simulink model "lab5_EAs"  (R2021b)
settings: Solver=VariableStepAuto  StartTime=0.0  StopTime=10.0  RelTol=1e-3
values from neighbouring files (symbols this model uses):
  J = [Ixx 0 0; 0 Iyy 0; 0 0 Izz]    [euler_equation_tasks.m]    (also in lab5_task2.m)
  Jinv = inv(J)    [euler_equation_tasks.m]    (also in lab5_task2.m)
  theta0 = deg2rad(0)    [Lab08_script.m]    (also in Lab7_script.m = deg2rad(230); Lab7_scriptscalar.m = deg2rad(230))
  w0 = [0.45 0.52 0.55]'    [euler_equation_tasks.m]    (also in lab5_task2.m = [C 0.1 0.1]')
undefined symbols (not defined in the file or in its folder): phi0, psi0
libraries: matrix_library x1
settings Model: Creator=samuz  LastModifiedBy=samuz

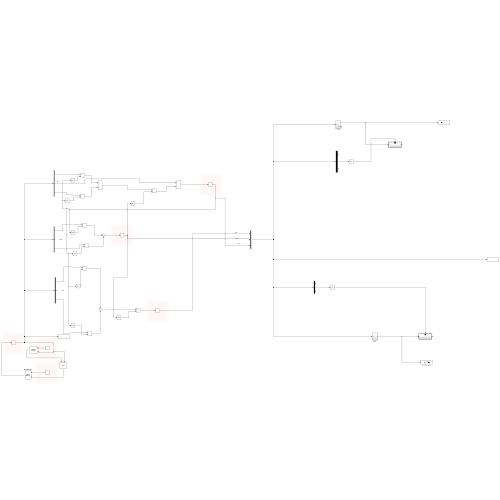
[thumbnail: Simulink's stored preview of the top-level diagram]
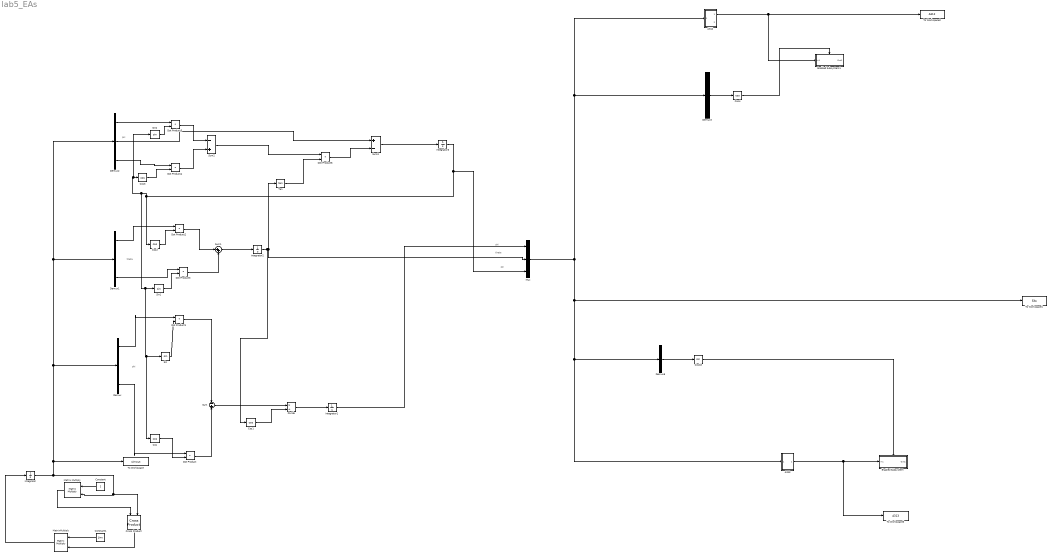
== system lab5_EAs ==
  note: psi
  note: theta
  note: phi
  note: psi
  note: theta
  note: phi
  A312 : Subsystem
  A313 : Subsystem
  Constant : Constant  Value=J
  Constant1 : Constant  Value=Jinv
  Cos{,1..4} (5 alike) : Trigonometry  Operator=cos
  Cos18 : Trigonometry
  Cross Product : matrix_library/Cross Product
      settings: SourceProductBaseCode=SL
  Demux{,1..3,6} (5 alike) : Demux  Outputs=3
  Divide : Product  Inputs=*/
  Dot Product{,1..6} (7 alike) : DotProduct  InputSameDT=on  OutDataTypeStr=Inherit: Inherit via internal rule
  Enabled Subsystem : Subsystem  TreatAsAtomicUnit=on
  Enabled Subsystem1 : Subsystem  TreatAsAtomicUnit=on
  Integrator : Integrator  InitialCondition=w0
  Integrator1 : Integrator  InitialCondition=phi0
  Integrator2 : Integrator  InitialCondition=theta0
  Integrator3 : Integrator  InitialCondition=psi0
  Matrix Multiply : Product  Multiplication=Matrix(*)
  MatrixMultiply : Product  Multiplication=Matrix(*)
  Mux : Mux  Inputs=3
  Sin : Trigonometry
  Sin1 : Trigonometry
  Sin2 : Trigonometry
  Sum : Sum  Inputs=-+
  Sum1 : Sum  Inputs=|++
  Sum2 : Sum  Inputs=-+
  Sum3 : Sum  Inputs=+-
  Tan : Trigonometry  Operator=tan
  To Workspace : ToWorkspace  VariableName=simout  SampleTime=-1
  To Workspace1 : ToWorkspace  VariableName=EAs  SampleTime=-1
  To Workspace2 : ToWorkspace  VariableName=A312  SaveFormat=Timeseries  SampleTime=-1
  To Workspace3 : ToWorkspace  VariableName=A313  SaveFormat=Timeseries  SampleTime=-1
  wires:
  Cross Product/1 -> MatrixMultiply/2
  Matrix Multiply/1 -> Cross Product/1
  Integrator/1 -> To Workspace/1, Demux2/1, Demux1/1, Demux/1, Cross Product/2, Matrix Multiply/2
  MatrixMultiply/1 -> Integrator/1
  Constant1/1 -> MatrixMultiply/1
  Constant/1 -> Matrix Multiply/1
  Demux/3 -> Dot Product/1
  Cos/1 -> Dot Product/2
  Demux/1 -> Dot Product1/1
  Sin/1 -> Dot Product1/2
  Dot Product1/1 -> Sum/1
  Dot Product/1 -> Sum/2
  Sum/1 -> Divide/1
  Cos1/1 -> Divide/2
  Divide/1 -> Integrator1/1
  Cos2/1 -> Dot Product2/2
  Sin1/1 -> Dot Product3/2
  Demux1/1 -> Dot Product2/1
  Demux1/3 -> Dot Product3/1
  Dot Product2/1 -> Sum1/1
  Dot Product3/1 -> Sum1/2
  Sum1/1 -> Integrator2/1
  Demux2/3 -> Dot Product4/1
  Cos3/1 -> Dot Product4/2
  Sin2/1 -> Dot Product5/2
  Demux2/1 -> Dot Product5/1
  Dot Product4/1 -> Sum2/2
  Dot Product5/1 -> Sum2/1
  Integrator2/1 -> Mux/2, Tan/1, Cos1/1
  Sum2/1 -> Dot Product6/1
  Tan/1 -> Dot Product6/2
  Dot Product6/1 -> Sum3/2
  Demux2/2 -> Sum3/1
  Sum3/1 -> Integrator3/1
  Integrator3/1 -> Cos/1, Sin/1, Sin1/1, Sin2/1, Cos3/1, Cos2/1, Mux/3
  Integrator1/1 -> Mux/1
  Mux/1 -> Demux3/1, A312/1(In1), Demux6/1, A313/1(In1), To Workspace1/1
  A313/1(Out1) -> Enabled Subsystem/1(In1), To Workspace3/1
  Demux6/2 -> Cos18/1
  Cos18/1 -> Enabled Subsystem/Enable
  A312/1(Out1) -> Enabled Subsystem1/1(In1), To Workspace2/1
  Demux3/2 -> Cos4/1
  Cos4/1 -> Enabled Subsystem1/Enable

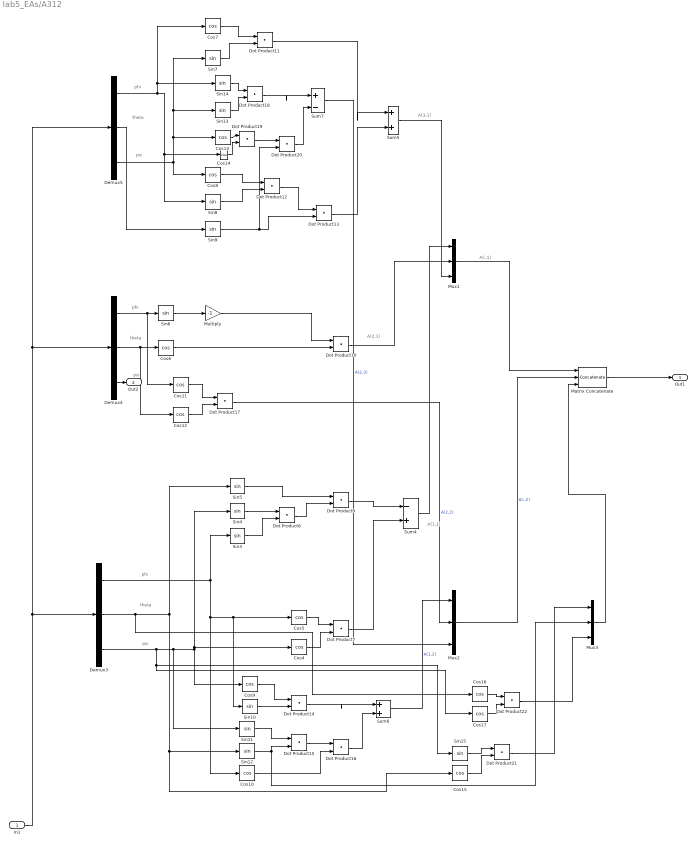
== system lab5_EAs/A312 ==
  note: A(:,1)
  note: A(3,1)
  note: A(2,1)
  note: A(1,1)
  note: psi
  note: psi
  note: theta
  note: phi
  note: phi
  note: theta
  note: psi
  note: phi
  note: theta
  In1 : Inport
  Cos{4..17} (14 alike) : Trigonometry  Operator=cos
  Demux3 : Demux  Outputs=3
  Demux4 : Demux  Outputs=3
  Demux5 : Demux  Outputs=3
  Dot Product{7..22} (16 alike) : DotProduct  InputSameDT=on  OutDataTypeStr=Inherit: Inherit via internal rule
  Matrix Concatenate : Concatenate  NumInputs=3  Mode=Multidimensional array  ConcatenateDimension=2
  Multiply : Gain  Gain=-1
  Mux1 : Mux  Inputs=3
  Mux2 : Mux  Inputs=3
  Mux3 : Mux  Inputs=3
  Sin{3..15} (13 alike) : Trigonometry
  Sum4 : Sum  Inputs=-+
  Sum5 : Sum  Inputs=|++
  Sum6 : Sum  Inputs=|++
  Sum7 : Sum  Inputs=|+-
  Out1 : Outport
  Out2 : Outport  Port=2
  wires:
  Cos15/1 -> Dot Product21/2
  Demux4/1 -> Cos11/1, Sin6/1
  Demux3/3 -> Cos17/1, Sin15/1, Sin11/1, Sin4/1, Cos4/1, Cos9/1
  Cos11/1 -> Dot Product17/1
  Sin11/1 -> Dot Product15/1
  Dot Product10/1 -> Mux1/2
  Demux5/3 -> Cos13/1, Sin7/1, Sin13/1, Cos8/1
  Sin7/1 -> Dot Product11/2
  Demux4/2 -> Cos12/1, Cos6/1
  Dot Product12/1 -> Dot Product13/1
  Dot Product7/1 -> Sum4/2
  Dot Product9/1 -> Sum4/1
  In1/1 -> Demux5/1, Demux4/1, Demux3/1
  Sin9/1 -> Dot Product20/2, Dot Product13/2
  Dot Product11/1 -> Sum5/1
  Sin10/1 -> Dot Product14/2
  Sin5/1 -> Dot Product9/1
  Dot Product15/1 -> Dot Product16/1
  Dot Product18/1 -> Sum7/1
  Sum5/1 -> Mux1/3
  Mux2/1 -> Matrix Concatenate/2  "A(:,2)"
  Demux5/1 -> Sin14/1, Cos7/1, Cos14/1, Sin8/1
  Sin3/1 -> Dot Product8/2
  Demux3/2 -> Cos16/1, Cos15/1, Sin12/1, Sin5/1
  Demux3/1 -> Cos10/1, Sin10/1, Cos5/1, Sin3/1
  Cos6/1 -> Dot Product10/2
  Cos7/1 -> Dot Product11/1
  Dot Product13/1 -> Sum5/2
  Sin6/1 -> Multiply/1
  Sin4/1 -> Dot Product8/1
  Dot Product22/1 -> Mux3/3
  Cos8/1 -> Dot Product12/1
  Multiply/1 -> Dot Product10/1
  Dot Product8/1 -> Dot Product9/2
  Demux4/3 -> Out2/1
  Cos5/1 -> Dot Product7/1
  Demux5/2 -> Sin9/1
  Sin15/1 -> Dot Product21/1
  Dot Product14/1 -> Sum6/1
  Cos10/1 -> Dot Product16/2
  Sin14/1 -> Dot Product18/1
  Sin13/1 -> Dot Product18/2
  Sum6/1 -> Mux2/1  "A(1,2)"
  Dot Product20/1 -> Sum7/2
  Sin8/1 -> Dot Product12/2
  Mux1/1 -> Matrix Concatenate/1
  Sum7/1 -> Mux2/3  "A(2,3)"
  Dot Product21/1 -> Mux3/1
  Cos12/1 -> Dot Product17/2
  Cos9/1 -> Dot Product14/1
  Sum4/1 -> Mux1/1
  Dot Product17/1 -> Mux2/2  "A(2,2)"
  Cos13/1 -> Dot Product19/1
  Cos14/1 -> Dot Product19/2
  Dot Product19/1 -> Dot Product20/1
  Cos16/1 -> Dot Product22/1
  Dot Product16/1 -> Sum6/2
  Cos4/1 -> Dot Product7/2
  Cos17/1 -> Dot Product22/2
  Sin12/1 -> Mux3/2, Dot Product15/2
  Mux3/1 -> Matrix Concatenate/3
  Matrix Concatenate/1 -> Out1/1

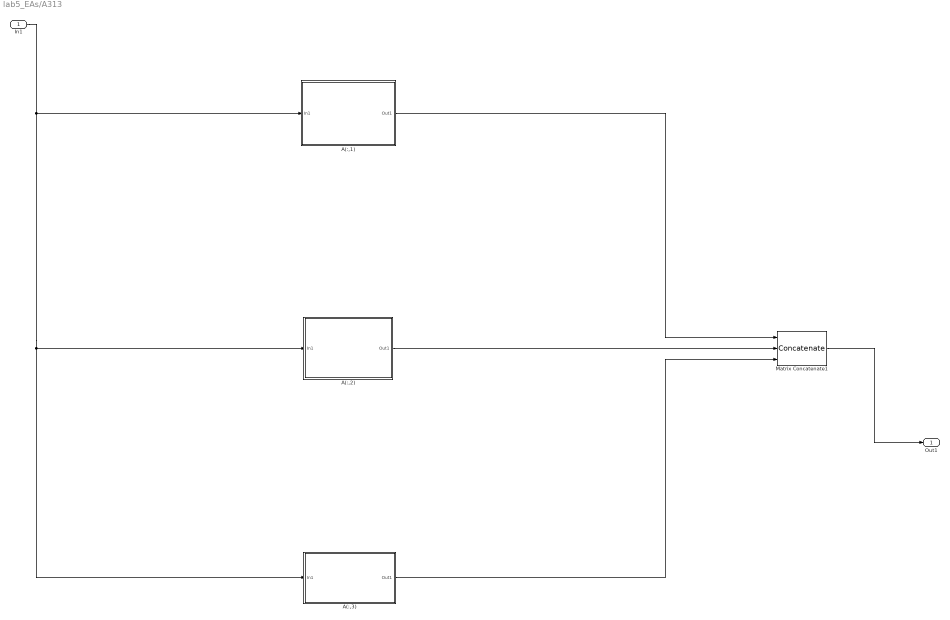
== system lab5_EAs/A313 ==
  In1 : Inport
  A(:,1) : Subsystem
  A(:,2) : Subsystem
  A(:,3) : Subsystem
  Matrix Concatenate1 : Concatenate  NumInputs=3  Mode=Multidimensional array  ConcatenateDimension=2
  Out1 : Outport
  wires:
  In1/1 -> A(:,3)/1(In1), A(:,2)/1(In1), A(:,1)/1(In1)
  A(:,3)/1(Out1) -> Matrix Concatenate1/3
  A(:,2)/1(Out1) -> Matrix Concatenate1/2
  A(:,1)/1(Out1) -> Matrix Concatenate1/1
  Matrix Concatenate1/1 -> Out1/1

== system lab5_EAs/Enabled Subsystem ==
  In1 : Inport
  Enable : EnablePort
  Out1 : Outport
  wires:
  In1/1 -> Out1/1

== system lab5_EAs/Enabled Subsystem1 ==
  In1 : Inport
  Enable : EnablePort
  Out1 : Outport
  wires:
  In1/1 -> Out1/1

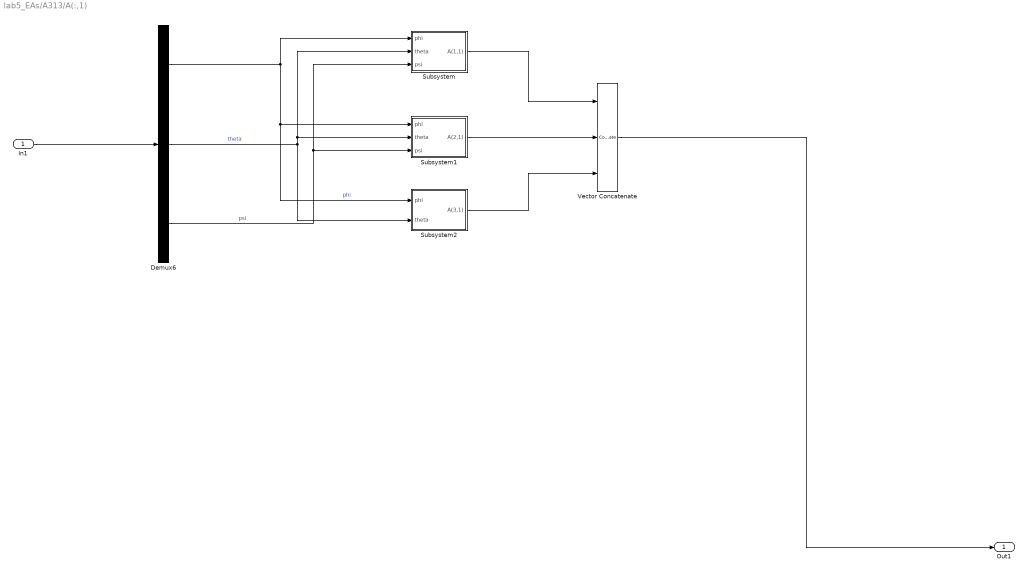
== system lab5_EAs/A313/A(:,1) ==
  In1 : Inport
  Demux6 : Demux  Outputs=3
  Subsystem : Subsystem
  Subsystem1 : Subsystem
  Subsystem2 : Subsystem
  Vector Concatenate : Concatenate  NumInputs=3
  Out1 : Outport
  wires:
  Subsystem2/1(A(3,1)) -> Vector Concatenate/3
  Demux6/1 -> Subsystem2/1(phi), Subsystem1/1(phi), Subsystem/1(phi)  "phi"
  Demux6/3 -> Subsystem1/3(psi), Subsystem/3(psi)  "psi"
  Subsystem1/1(A(2,1)) -> Vector Concatenate/2
  Demux6/2 -> Subsystem2/2(theta), Subsystem1/2(theta), Subsystem/2(theta)  "theta"
  In1/1 -> Demux6/1
  Subsystem/1(A(1,1)) -> Vector Concatenate/1
  Vector Concatenate/1 -> Out1/1

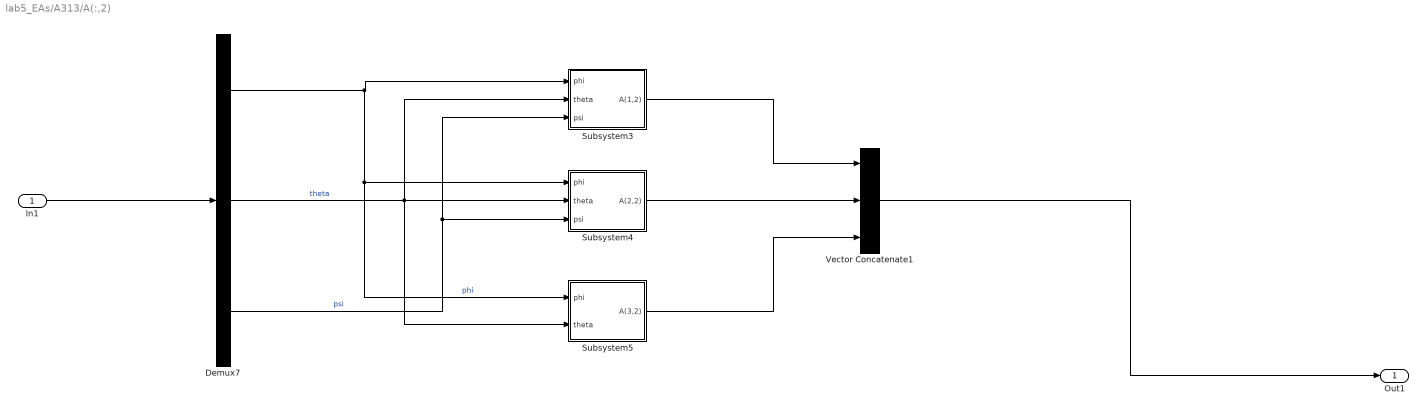
== system lab5_EAs/A313/A(:,2) ==
  In1 : Inport
  Demux7 : Demux  Outputs=3
  Subsystem3 : Subsystem
  Subsystem4 : Subsystem
  Subsystem5 : Subsystem
  Vector Concatenate1 : Concatenate  NumInputs=3
  Out1 : Outport
  wires:
  Demux7/3 -> Subsystem4/3(psi), Subsystem3/3(psi)  "psi"
  Subsystem5/1(A(3,2)) -> Vector Concatenate1/3
  In1/1 -> Demux7/1
  Subsystem4/1(A(2,2)) -> Vector Concatenate1/2
  Demux7/1 -> Subsystem3/1(phi), Subsystem5/1(phi), Subsystem4/1(phi)  "phi"
  Vector Concatenate1/1 -> Out1/1
  Demux7/2 -> Subsystem4/2(theta), Subsystem5/2(theta), Subsystem3/2(theta)  "theta"
  Subsystem3/1(A(1,2)) -> Vector Concatenate1/1

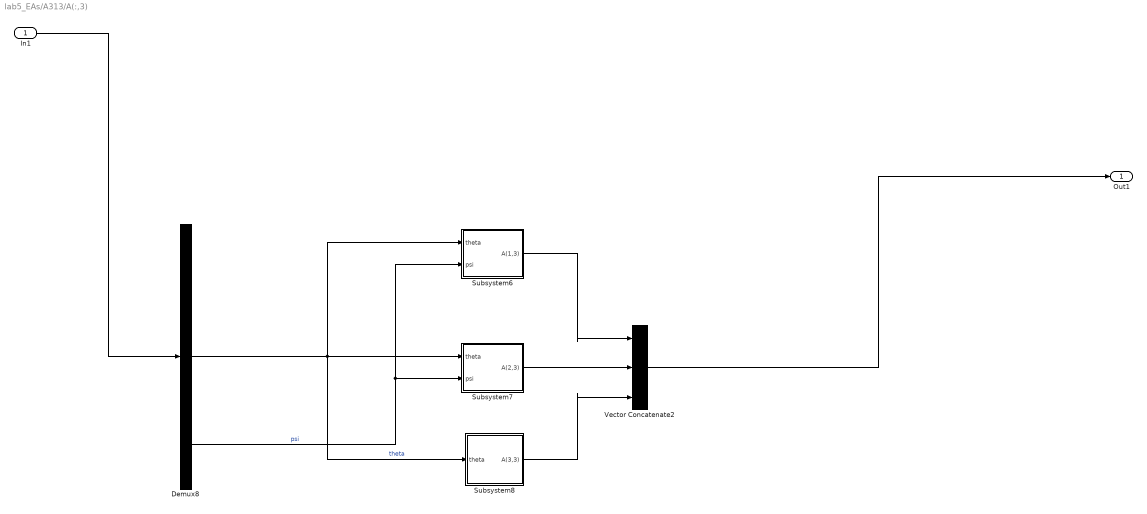
== system lab5_EAs/A313/A(:,3) ==
  In1 : Inport
  Demux8 : Demux  Outputs=3
  Subsystem6 : Subsystem
  Subsystem7 : Subsystem
  Subsystem8 : Subsystem
  Vector Concatenate2 : Concatenate  NumInputs=3
  Out1 : Outport
  wires:
  Demux8/2 -> Subsystem8/1(theta), Subsystem6/1(theta), Subsystem7/1(theta)  "theta"
  Subsystem7/1(A(2,3)) -> Vector Concatenate2/2
  Vector Concatenate2/1 -> Out1/1
  Subsystem8/1(A(3,3)) -> Vector Concatenate2/3
  Subsystem6/1(A(1,3)) -> Vector Concatenate2/1
  In1/1 -> Demux8/1
  Demux8/3 -> Subsystem7/2(psi), Subsystem6/2(psi)  "psi"

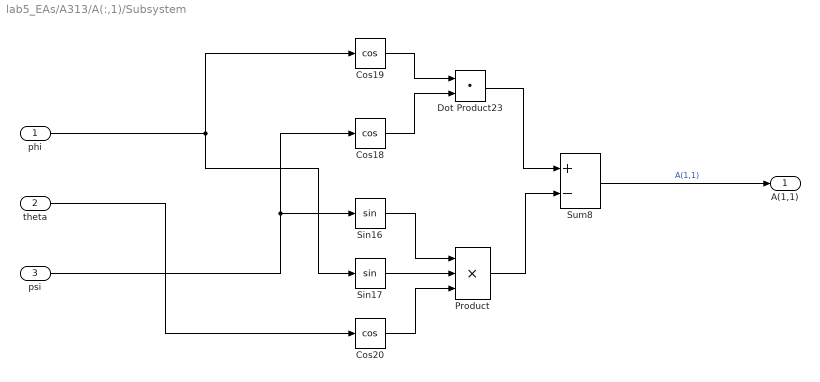
== system lab5_EAs/A313/A(:,1)/Subsystem ==
  phi : Inport
  theta : Inport  Port=2
  psi : Inport  Port=3
  Cos18 : Trigonometry  Operator=cos
  Cos19 : Trigonometry  Operator=cos
  Cos20 : Trigonometry  Operator=cos
  Dot Product23 : DotProduct  InputSameDT=on  OutDataTypeStr=Inherit: Inherit via internal rule
  Product : Product  Inputs=3
  Sin16 : Trigonometry
  Sin17 : Trigonometry
  Sum8 : Sum  Inputs=+-
  A(1,1) : Outport
  wires:
  psi/1 -> Sin16/1, Cos18/1
  Dot Product23/1 -> Sum8/1
  Sin16/1 -> Product/1
  Cos18/1 -> Dot Product23/2
  Sin17/1 -> Product/2
  Cos19/1 -> Dot Product23/1
  Product/1 -> Sum8/2
  Sum8/1 -> A(1,1)/1  "A(1,1)"
  Cos20/1 -> Product/3
  phi/1 -> Cos19/1, Sin17/1
  theta/1 -> Cos20/1

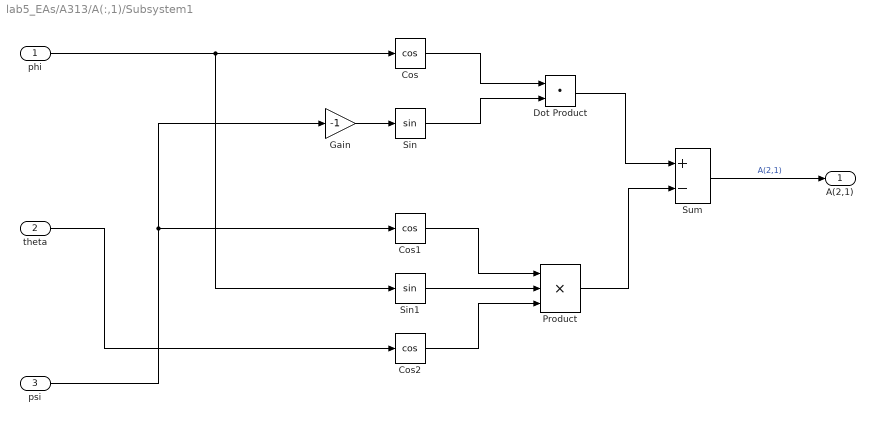
== system lab5_EAs/A313/A(:,1)/Subsystem1 ==
  phi : Inport
  theta : Inport  Port=2
  psi : Inport  Port=3
  Cos : Trigonometry  Operator=cos
  Cos1 : Trigonometry  Operator=cos
  Cos2 : Trigonometry  Operator=cos
  Dot Product : DotProduct  InputSameDT=on  OutDataTypeStr=Inherit: Inherit via internal rule
  Gain : Gain  Gain=-1
  Product : Product  Inputs=3
  Sin : Trigonometry
  Sin1 : Trigonometry
  Sum : Sum  Inputs=+-
  A(2,1) : Outport
  wires:
  psi/1 -> Cos1/1, Gain/1
  phi/1 -> Cos/1, Sin1/1
  Gain/1 -> Sin/1
  Cos/1 -> Dot Product/1
  Sin/1 -> Dot Product/2
  theta/1 -> Cos2/1
  Cos1/1 -> Product/1
  Sin1/1 -> Product/2
  Cos2/1 -> Product/3
  Dot Product/1 -> Sum/1
  Product/1 -> Sum/2
  Sum/1 -> A(2,1)/1  "A(2,1)"

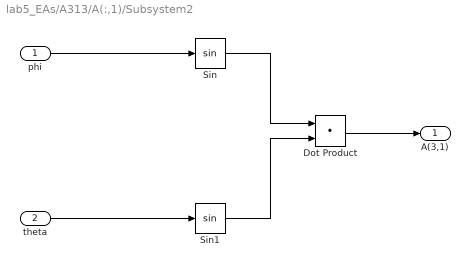
== system lab5_EAs/A313/A(:,1)/Subsystem2 ==
  phi : Inport
  theta : Inport  Port=2
  Dot Product : DotProduct  InputSameDT=on  OutDataTypeStr=Inherit: Inherit via internal rule
  Sin : Trigonometry
  Sin1 : Trigonometry
  A(3,1) : Outport
  wires:
  phi/1 -> Sin/1
  theta/1 -> Sin1/1
  Sin/1 -> Dot Product/1
  Sin1/1 -> Dot Product/2
  Dot Product/1 -> A(3,1)/1

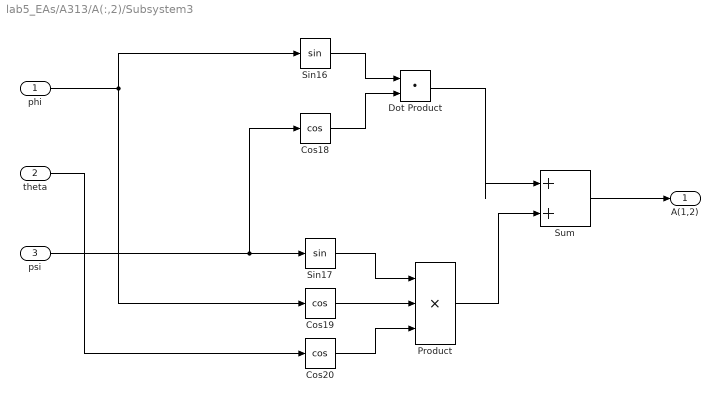
== system lab5_EAs/A313/A(:,2)/Subsystem3 ==
  phi : Inport
  theta : Inport  Port=2
  psi : Inport  Port=3
  Cos18 : Trigonometry  Operator=cos
  Cos19 : Trigonometry  Operator=cos
  Cos20 : Trigonometry  Operator=cos
  Dot Product : DotProduct  InputSameDT=on  OutDataTypeStr=Inherit: Inherit via internal rule
  Product : Product  Inputs=3
  Sin16 : Trigonometry
  Sin17 : Trigonometry
  Sum : Sum  Inputs=|++
  A(1,2) : Outport
  wires:
  Cos18/1 -> Dot Product/2
  phi/1 -> Cos19/1, Sin16/1
  psi/1 -> Cos18/1, Sin17/1
  Sin16/1 -> Dot Product/1
  theta/1 -> Cos20/1
  Sin17/1 -> Product/1
  Cos19/1 -> Product/2
  Cos20/1 -> Product/3
  Dot Product/1 -> Sum/1
  Product/1 -> Sum/2
  Sum/1 -> A(1,2)/1

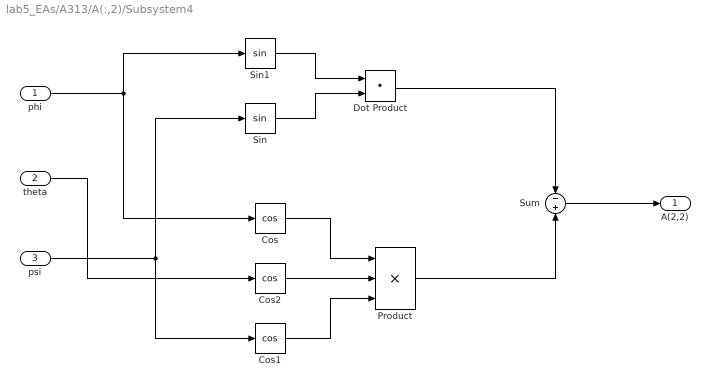
== system lab5_EAs/A313/A(:,2)/Subsystem4 ==
  phi : Inport
  theta : Inport  Port=2
  psi : Inport  Port=3
  Cos : Trigonometry  Operator=cos
  Cos1 : Trigonometry  Operator=cos
  Cos2 : Trigonometry  Operator=cos
  Dot Product : DotProduct  InputSameDT=on  OutDataTypeStr=Inherit: Inherit via internal rule
  Product : Product  Inputs=3
  Sin : Trigonometry
  Sin1 : Trigonometry
  Sum : Sum  Inputs=-+
  A(2,2) : Outport
  wires:
  phi/1 -> Sin1/1, Cos/1
  psi/1 -> Cos1/1, Sin/1
  Sin1/1 -> Dot Product/1
  Sin/1 -> Dot Product/2
  theta/1 -> Cos2/1
  Cos2/1 -> Product/2
  Cos/1 -> Product/1
  Cos1/1 -> Product/3
  Dot Product/1 -> Sum/1
  Product/1 -> Sum/2
  Sum/1 -> A(2,2)/1

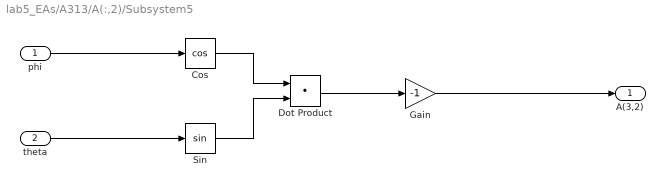
== system lab5_EAs/A313/A(:,2)/Subsystem5 ==
  phi : Inport
  theta : Inport  Port=2
  Cos : Trigonometry  Operator=cos
  Dot Product : DotProduct  InputSameDT=on  OutDataTypeStr=Inherit: Inherit via internal rule
  Gain : Gain  Gain=-1
  Sin : Trigonometry
  A(3,2) : Outport
  wires:
  phi/1 -> Cos/1
  theta/1 -> Sin/1
  Cos/1 -> Dot Product/1
  Sin/1 -> Dot Product/2
  Dot Product/1 -> Gain/1
  Gain/1 -> A(3,2)/1

== system lab5_EAs/A313/A(:,3)/Subsystem6 ==
  theta : Inport
  psi : Inport  Port=2
  Dot Product : DotProduct  InputSameDT=on  OutDataTypeStr=Inherit: Inherit via internal rule
  Sin : Trigonometry
  Sin1 : Trigonometry
  A(1,3) : Outport
  wires:
  psi/1 -> Sin/1
  theta/1 -> Sin1/1
  Dot Product/1 -> A(1,3)/1
  Sin1/1 -> Dot Product/1
  Sin/1 -> Dot Product/2

== system lab5_EAs/A313/A(:,3)/Subsystem7 ==
  theta : Inport
  psi : Inport  Port=2
  Dot Product : DotProduct  InputSameDT=on  OutDataTypeStr=Inherit: Inherit via internal rule
  Sin : Trigonometry  Operator=cos
  Sin1 : Trigonometry
  A(2,3) : Outport
  wires:
  psi/1 -> Sin/1
  theta/1 -> Sin1/1
  Dot Product/1 -> A(2,3)/1
  Sin1/1 -> Dot Product/1
  Sin/1 -> Dot Product/2

== system lab5_EAs/A313/A(:,3)/Subsystem8 ==
  theta : Inport
  Cos18 : Trigonometry  Operator=cos
  A(3,3) : Outport
  wires:
  theta/1 -> Cos18/1
  Cos18/1 -> A(3,3)/1
